simulink model "L_detector"  (Simulink 7.6)
settings: Solver=FixedStepDiscrete  StartTime=0.0  StopTime=0  RelTol=1e-3
undefined symbols (not defined in the file or in its folder): Rec, SDTV
libraries: vipconversions x1, vipanalysis x1, viptransforms x1
settings Model: Creator=Thing 1  LastModifiedBy=Administrator
settings RTWCC: TargetLang=C++

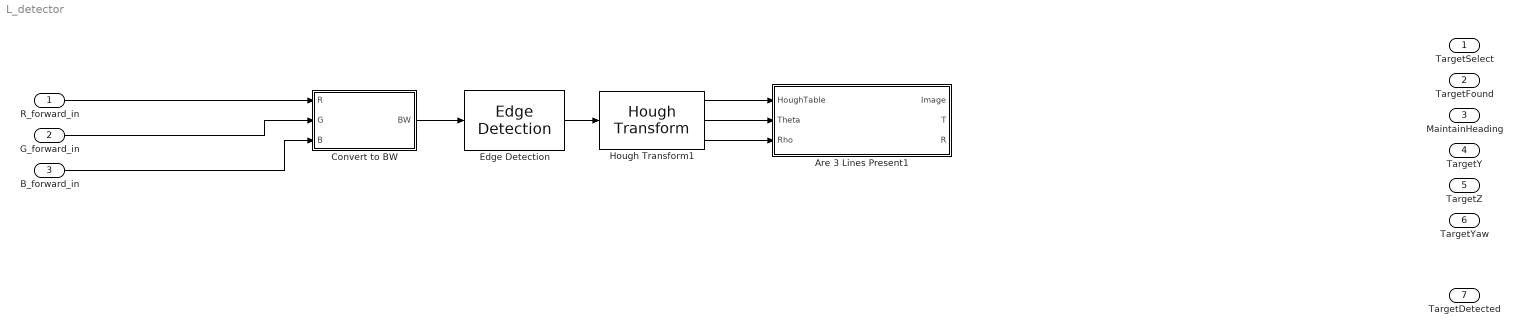
== system L_detector ==
  R_forward_in : Inport  PortDimensions=[120 160]
  G_forward_in : Inport  Port=2  PortDimensions=[120 160]
  B_forward_in : Inport  Port=3  PortDimensions=[120 160]
  Are 3 Lines Present1 : Stateflow chart  TreatAsAtomicUnit=on  SystemSampleTime=[1/30 0]
  Convert to BW : Subsystem
  Edge Detection : vipanalysis/Edge Detection  DialogController=vipDDGCreate  DialogControllerArgs=DataTag0  method=Sobel  outputType=Binary image  userDefinedThreshold=off  thresholdSource=Specify via dialog  threshold=20  thresholdTuning=3  edgeThinning=on  threshold_canny=[0.25 0.60]  autoPercent=70  sigma=1  roundingMode=Floor  overflowMode=off
  Hough Transform1 : viptransforms/Hough Transform  DialogController=vipDDGCreate  DialogControllerArgs=DataTag1  theta_res=pi/180  rho_res=1  out_theta_rho=on  outdtmode=double  firstCoeffMode=Binary point scaling  firstCoeffWordLength=16  firstCoeffFracLength=14  secondCoeffMode=Binary point scaling  secondCoeffWordLength=32  secondCoeffFracLength=16  outputMode=Binary point scaling  outputWordLength=16  outputFracLength=0  accumMode=Binary point scaling  accumWordLength=32  accumFracLength=20  prodOutputMode=Binary point scaling  prodOutputWordLength=32  prodOutputFracLength=20  memoryMode=Binary point scaling  memoryWordLength=32  memoryFracLength=16  roundingMode=Nearest  overflowMode=on
  TargetSelect : Outport  OutDataTypeStr=double
  TargetFound : Outport  Port=2  OutDataTypeStr=double
  MaintainHeading : Outport  Port=3  OutDataTypeStr=double
  TargetY : Outport  Port=4  OutDataTypeStr=double
  TargetZ : Outport  Port=5  OutDataTypeStr=double
  TargetYaw : Outport  Port=6  OutDataTypeStr=double
  TargetDetected : Outport  Port=7  OutDataTypeStr=double
  wires:
  Convert to BW/1(BW) -> Edge Detection/1
  Hough Transform1/1 -> Are 3 Lines Present1/1(HoughTable)
  Hough Transform1/2 -> Are 3 Lines Present1/2(Theta)
  Hough Transform1/3 -> Are 3 Lines Present1/3(Rho)
  Edge Detection/1 -> Hough Transform1/1
  G_forward_in/1 -> Convert to BW/2(G)
  R_forward_in/1 -> Convert to BW/1(R)
  B_forward_in/1 -> Convert to BW/3(B)

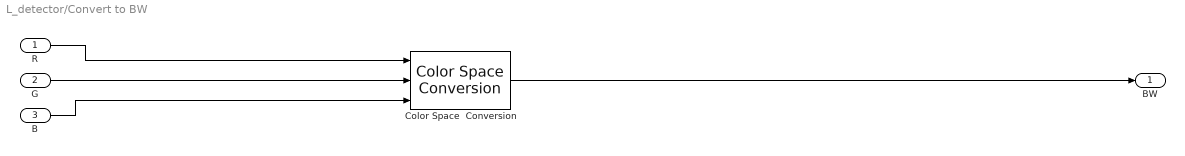
== system L_detector/Convert to BW ==
  R : Inport  OutDataTypeStr=double
  G : Inport  Port=2  OutDataTypeStr=double
  B : Inport  Port=3  OutDataTypeStr=double
  Color Space  Conversion : vipconversions/Color Space  Conversion  conversion=Obsolete  conversionActive=R'G'B' to intensity  wp_str=D65  rec=Rec. 601 (SDTV)  sys=1125/60/2:1  imagePorts=Separate color signals
  BW : Outport
  wires:
  R/1 -> Color Space  Conversion/1
  G/1 -> Color Space  Conversion/2
  B/1 -> Color Space  Conversion/3
  Color Space  Conversion/1 -> BW/1

== matlab function Are 3 Lines Present1 ==
  data: HoughTable input double; Image output double; T output double; Theta input double; Rho input double; R output double
function [Image,T,R] = AreLinesPresent(HoughTable,Theta,Rho)
% This function is meant to see if there are 3 lines which approximate a
% 'hedge' in the current frame

R = zeros(1,2);
T = zeros(1,2);
[rhos, thetas] = size(HoughTable);

% Find the two vetical lines
theta_0_col = floor(thetas/2);

most_votes = 0;
second_most = 0;
indexi1 = 1;
indexi2 = 1;
indexj1 = 1;
indexj2 = 1;


for i = 1:rhos
    for j = theta_0_col-5:theta_0_col+5
        if(HoughTable(i,j) > most_votes)
            %{
            if(abs(Rho(indexi1)-Rho(i)) > 20)
                second_most = HoughTable(indexi1,indexj2);
                indexi2 = indexi1;
                indexj2 = indexj1;
                R(2) = R(1);
                T(2) = T(1);
            end
            %}
            most_votes = HoughTable(i,j);
            indexi1 = i;
            indexj1 = j;
            R(1) = Rho(i);
            T(1) = Theta(j);
        %{
elseif(HoughTable(i,j) > second_most && abs(Rho(indexi1)-Rho(i)) > 20)
            second_most = HoughTable(i,j);
            indexi2 = i;
            indexj2 = j;
            R(2) = Rho(i);
            T(2) = Theta(j);
%}
        end
    end
end

% Find the horizontal line
max_votes = 0;
index = [0 0];
for i = 1:rhos
    for j = 1:10
        if(HoughTable(i,j) > max_votes)
            max_votes = HoughTable(i,j);
            index = [i,j];
            R(2) = Rho(i);
            T(2) = Theta(j);
        end
    end
    for j = thetas-10:thetas
        if(HoughTable(i,j) > max_votes)
            max_votes = HoughTable(i,j);
            index = [i,j];
            R(2) = Rho(i);
            T(2) = Theta(j);
        end
    end
end

% Find the most prominent line
top_vote = 0;
t = 0;
r = 0;
for i = 1:rhos
    for j = 1:thetas
        if(HoughTable(i,j) > top_vote)
            top_vote = HoughTable(i,j);
            t = j;
            r = i;
        end
    end
end

Image = 0;
if(top_vote*.75 < max_votes && top_vote*.3 < most_votes && top_vote*.3 < second_most)
    Image = 1;
end

cow = 1;

return
